simulink library "mixer_lib"  (Simulink 8.7)
settings: Solver=ode45  StartTime=0.0  StopTime=10.0  RelTol=1e-3
undefined symbols (not defined in the file): AdvDSPBChannelOutDisplay, DDC_CM_multiplication_factor, DDC_CM_NCO_phase, DDC_CM_NCO_sync, DDC_CM_number_of_bits_to_shift_left, DDC_LINEUP_param, dpoly, dspba_ChannelInVis, dspba_ChannelOutVis, dspba_internal_get_channel_ports, latency, value
libraries: DSPBAPrim x6, DSPBAWaveformSynth x2, DSPBABase x1
Description:
  | Digital Down Conversion 4 channel, 4 antenna reference design - complex mixer library
settings Model: Creator=bigcat  LastModifiedBy=5g

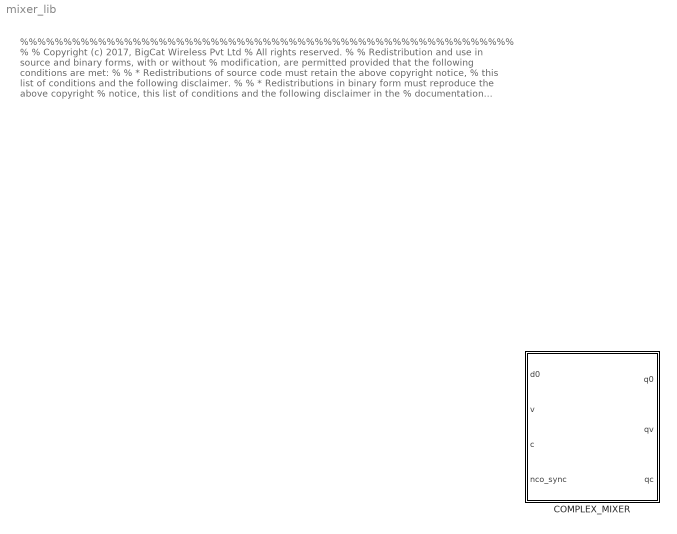
== system mixer_lib ==
  note: %%%%%%%%%%%%%%%%%%%%%%%%%%%%%%%%%%%%%%%%%%%%%%%%%%%%%%%%%
      |  %
      |  % Copyright (c) 2017, BigCat Wireless Pvt Ltd
      |  % All rights reserved.
      |  %
      |  % Redistribution and use in source and binary forms, with or without
      |  % modification, are permitted provided that the following conditions are met:
      |  %
      |  %     * Redistributions of source code must retain the above copyright notice,
      |  %       this list of conditions and the following disclaimer.
      |  %
      |  %     * Redistributions in binary form must reproduce the above copyright
      |  %       notice, this list of conditions and the following disclaimer in the
      |  %       documentation and/or other materials provided with the distribution.
      |  %
      |  %     * Neither the name of the copyright holder nor the names of its contributors
      |  %       may be used to endorse or promote products derived from this software
      |  %       without specific prior written permission.
      |  %
      |  %
      |  %
      |  % THIS SOFTWARE IS PROVIDED BY THE COPYRIGHT HOLDERS AND CONTRIBUTORS "AS IS"
      |  % AND ANY EXPRESS OR IMPLIED WARRANTIES, INCLUDING, BUT NOT LIMITED TO, THE
      |  % IMPLIED WARRANTIES OF MERCHANTABILITY AND FITNESS FOR A PARTICULAR PURPOSE ARE
      |  % DISCLAIMED. IN NO EVENT SHALL THE COPYRIGHT HOLDER OR CONTRIBUTORS BE LIABLE
      |  % FOR ANY DIRECT, INDIRECT, INCIDENTAL, SPECIAL, EXEMPLARY, OR CONSEQUENTIAL
      |  % DAMAGES (INCLUDING, BUT NOT LIMITED TO, PROCUREMENT OF SUBSTITUTE GOODS OR
      |  % SERVICES; LOSS OF USE, DATA, OR PROFITS; OR BUSINESS INTERRUPTION) HOWEVER
      |  % CAUSED AND ON ANY THEORY OF LIABILITY, WHETHER IN CONTRACT, STRICT LIABILITY,
      |  % OR TORT (INCLUDING NEGLIGENCE OR OTHERWISE) ARISING IN ANY WAY OUT OF THE USE
      |  % OF THIS SOFTWARE, EVEN IF ADVISED OF THE POSSIBILITY OF SUCH DAMAGE.
      |  %
      |   %%%%%%%%%%%%%%%%%%%%%%%%%%%%%%%%%%%%%%%%%%%%%%%%%%%%%%%%%%
  COMPLEX_MIXER : Subsystem  mask{CM_clock_margin=DDC_LINEUP_param.ClockMargin, CM_NCO_sample_rate=DDC_LINEUP_param.Complex_NCO.sample_rate, CM_NCO_accumulator_bit_width=DDC_LINEUP_param.Complex_NCO.accum_bit_width, CM_NCO_frequency_word=DDC_LINEUP_param.Complex_NCO.freq_word, CM_NCO_base_addr=DDC_LINEUP_param.Complex_NCO.base_addr, CM_NCO_data_type=DDC_LINEUP_param.Complex_NCO.data_type, CM_NCO_scaling_value=DDC_LINEUP_param.Complex_NCO.scaling_value, CM_sample_rate=DDC_LINEUP_param.CM.SampleRate, CM_complex_channels=DDC_LINEUP_param.CM.num_complex_chans, CM_complex_freq=DDC_LINEUP_param.CM.num_complex_freqs, CM_output_word_length=DDC_LINEUP_param.output_word_length, CM_output_fraction_length=DDC_LINEUP_param.output_fraction_length, CM_scale_multiplication_factor=DDC_CM_multiplication_factor, CM_scale_left_shift_factor=DDC_CM_number_of_bits_to_shift_left, CM_NCO_phase=DDC_CM_NCO_phase, CM_NCO_sync=DDC_CM_NCO_sync}
      mask prompts: CM_clock_margin "Clock margin"; CM_NCO_sample_rate "NCO sample rate"; CM_NCO_accumulator_bit_width "NCO accumulator bit width"; CM_NCO_frequency_word "NCO Frequency word"; CM_NCO_base_addr "NCO base address"; CM_NCO_data_type "NCO data type"; CM_NCO_scaling_value "NCO scaling value"; CM_sample_rate "Sample Rate"; CM_complex_channels "Number of complex channels"; CM_complex_freq "Number of complex frequencies"; CM_output_word_length "Output word length"; CM_output_fraction_length "Output fraction length"; CM_scale_multiplication_factor "Scale multiplication factor"; CM_scale_left_shift_factor "Scale left-shift factor"; CM_NCO_phase "NCO phase"; CM_NCO_sync "NCO sync"
      mask Display:
      | disp('COMPLEX\nMIXER');
      | port_label('input',1,'d0');
      | port_label('input',2,'v');
      | port_label('input',3,'c');
      | port_label('input',4,'nco_sync');
      | port_label('output',1,'q0');
      | port_label('output',2,'qv');
      | port_label('output',3,'qc');

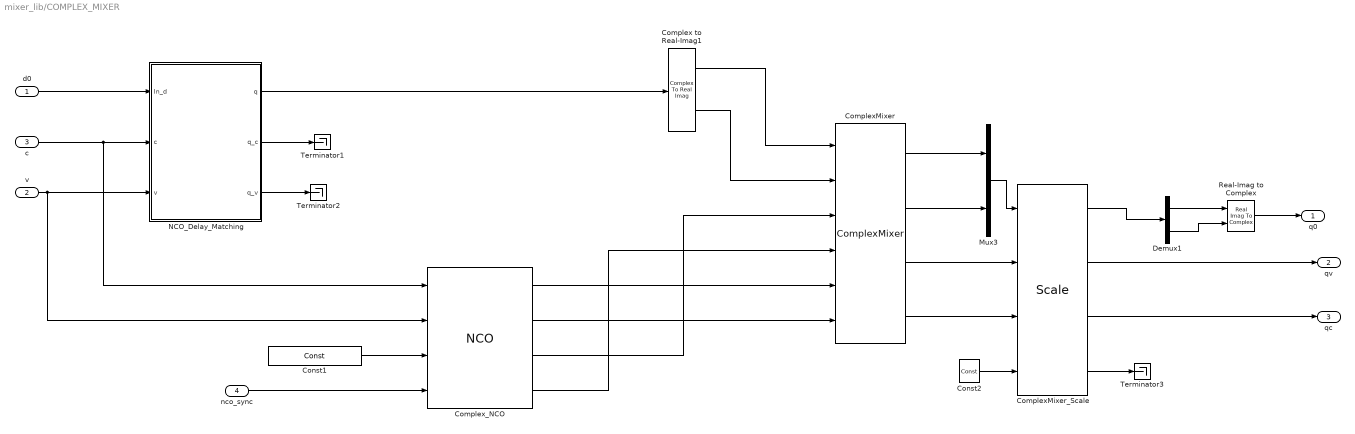
== system mixer_lib/COMPLEX_MIXER ==
  d0 : Inport
  v : Inport  Port=2
  c : Inport  Port=3
  nco_sync : Inport  Port=4
  Complex to Real-Imag1 : ComplexToRealImag
  ComplexMixer : DSPBAWaveformSynth/ComplexMixer  nInputRate=CM_sample_rate  nchan=CM_complex_channels  nfreq=CM_complex_freq  latency=4  version=20090407
  ComplexMixer_Scale : DSPBABase/Scale  otype=sfix(CM_output_word_length)  scale=2^-CM_output_fraction_length  rndmethod=Truncate  factor=CM_scale_multiplication_factor  satmethod=None  shift_vec=CM_scale_left_shift_factor  latency=0  wideSimulation=off  version=20130807
  Complex_NCO : DSPBAWaveformSynth/NCO  outputRate=CM_NCO_sample_rate  otype=sfix(CM_NCO_data_type)  scale=2^-CM_NCO_scaling_value  expSFDR=96.32  accumBitWidth=CM_NCO_accumulator_bit_width  accumPrecision=+/- 3.6621  phaseIncrAndInv=CM_NCO_frequency_word  phaseIncrInMHz="[0  0  0  0  0  0  0  0]"  phaseIncrAndInvMap=CM_NCO_base_addr  rwmode=Read/Write  exposebus=off  outWidth=5  tableSize=8  latency=18  version=20090407
      settings: AttributesFormatString=%<latency>
  Const1 : DSPBAPrim/Const  primtype=const  nInputs=0  nOutputs=1  omode=Specify via dialog  otype=ufix(24)  scale=2^-0  rndmethod=Unbiased  factor=1  satmethod=Symmetric  shift_vec=[0 1 2 -1]  value=CM_NCO_phase  inPortNames=['+'; '+';]  outPortNames=[' ']  dspbaimage=dspba_prim.jpg  text=fprintf('%s', num2str(value));  style=Optimised  visibilities=8 + 1024  floatPrecision=float32_m23  version=20120820
  Const2 : DSPBAPrim/Const  primtype=const  nInputs=0  nOutputs=1  omode=Specify via dialog  otype=ufix(1)  scale=1  rndmethod=Unbiased  factor=1  satmethod=Symmetric  shift_vec=[0 1 2 -1]  value=0  inPortNames=['+'; '+';]  outPortNames=[' ']  dspbaimage=dspba_prim.jpg  text=fprintf('%s', num2str(value));  style=Optimised  visibilities=8 + 1024  floatPrecision=float32_m23  version=20120820
  Demux1 : Demux  Outputs=2
  Mux3 : Mux  Inputs=2
  "NCO_Delay_Matching " : Subsystem
  Real-Imag to Complex : RealImagToComplex
  Terminator1 : Terminator
  Terminator2 : Terminator
  Terminator3 : Terminator
  q0 : Outport
  qv : Outport  Port=2
  qc : Outport  Port=3
  wires:
  Demux1/2 -> Real-Imag to Complex/2
  Demux1/1 -> Real-Imag to Complex/1
  ComplexMixer_Scale/4 -> Terminator3/1
  Const2/1 -> ComplexMixer_Scale/4
  Complex_NCO/1 -> ComplexMixer/5
  Complex_NCO/2 -> ComplexMixer/6
  ComplexMixer_Scale/3 -> qc/1
  ComplexMixer_Scale/2 -> qv/1
  ComplexMixer/1 -> Mux3/1
  ComplexMixer/2 -> Mux3/2
  Mux3/1 -> ComplexMixer_Scale/1
  ComplexMixer/4 -> ComplexMixer_Scale/3
  ComplexMixer/3 -> ComplexMixer_Scale/2
  Const1/1 -> Complex_NCO/3
  Real-Imag to Complex/1 -> q0/1
  ComplexMixer_Scale/1 -> Demux1/1
  Complex to Real-Imag1/1 -> ComplexMixer/1
  Complex_NCO/4 -> ComplexMixer/4
  Complex_NCO/3 -> ComplexMixer/3
  Complex to Real-Imag1/2 -> ComplexMixer/2
  "NCO_Delay_Matching "/1(q) -> Complex to Real-Imag1/1
  "NCO_Delay_Matching "/2(q_c) -> Terminator1/1
  "NCO_Delay_Matching "/3(q_v) -> Terminator2/1
  d0/1 -> "NCO_Delay_Matching "/1(In_d)
  c/1 -> Complex_NCO/1, "NCO_Delay_Matching "/2(c)
  v/1 -> Complex_NCO/2, "NCO_Delay_Matching "/3(v)
  nco_sync/1 -> Complex_NCO/4

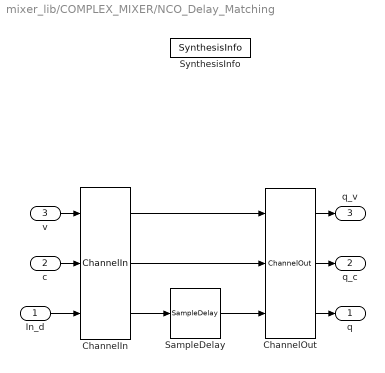
== system mixer_lib/COMPLEX_MIXER/NCO_Delay_Matching  ==
  In_d : Inport
  c : Inport  Port=2
  v : Inport  Port=3
  ChannelIn : DSPBAPrim/ChannelIn  primtype=channelin  nInputs=dspba_internal_get_channel_ports(gcb)  nOutputs=dspba_internal_get_channel_ports(gcb)  omode=Inherit via internal rule  otype=sfix(16)  scale=2^-15  rndmethod=Unbiased  factor=1  satmethod=Symmetric  shift_vec=[0 1 2 -1]  value=1  inPortNames=['v'; 'c'; '0'; '1'; '2'; '3'; '4'; '5'; '6'; '7'; '8'; '9'; 'A'; 'B'; 'D'; 'E'; 'F'; 'G'; 'H'; 'I'; 'J'; 'K'; 'L'; 'M'; 'N'; 'O'; 'P'; 'Q'; 'R'; 'S'; 'T'; 'U'; 'W'; 'X'; 'Y'; 'Z']  outPortNames=['v'; 'c'; '0'; '1'; '2'; '3'; '4'; '5'; '6'; '7'; '8'; '9'; 'A'; 'B'; 'D'; 'E'; 'F'; 'G'; 'H'; 'I'; 'J'; 'K'; 'L'; 'M'; 'N'; 'O'; 'P'; 'Q'; 'R'; 'S'; 'T'; 'U'; 'W'; 'X'; 'Y'; 'Z']  dspbaimage=dspba_prim.jpg  text=fprintf('In');  style=Optimised  dataSignals=1  foldingEnabled=off  channels=1  sampleRate=200  packetBeginPresent=off  packetBeginEnabled=off  visibilities=dspba_ChannelInVis(gcb)  latencyCorrection=0  version=20141013
  ChannelOut : DSPBAPrim/ChannelOut  primtype=channelout  nInputs=dspba_internal_get_channel_ports(gcb)  nOutputs=dspba_internal_get_channel_ports(gcb)  omode=Inherit via internal rule  otype=sfix(16)  scale=2^-15  rndmethod=Unbiased  factor=1  satmethod=Symmetric  shift_vec=[0 1 2 -1]  value=1  inPortNames=['v'; 'c'; '0'; '1'; '2'; '3'; '4'; '5'; '6'; '7'; '8'; '9'; 'A'; 'B'; 'D'; 'E'; 'F'; 'G'; 'H'; 'I'; 'J'; 'K'; 'L'; 'M'; 'N'; 'O'; 'P'; 'Q'; 'R'; 'S'; 'T'; 'U'; 'W'; 'X'; 'Y'; 'Z']  outPortNames=['v'; 'c'; '0'; '1'; '2'; '3'; '4'; '5'; '6'; '7'; '8'; '9'; 'A'; 'B'; 'D'; 'E'; 'F'; 'G'; 'H'; 'I'; 'J'; 'K'; 'L'; 'M'; 'N'; 'O'; 'P'; 'Q'; 'R'; 'S'; 'T'; 'U'; 'W'; 'X'; 'Y'; 'Z']  dspbaimage=dspba_prim.jpg  text=fprintf('Out%s', AdvDSPBChannelOutDisplay(latency));  style=Optimised  dataSignals=1  foldingEnabled=off  channels=1  sampleRate=200  packetBeginPresent=off  packetBeginEnabled=off  visibilities=dspba_ChannelOutVis(gcb)  latency=0  latencyCorrection=0  version=20141013
  SampleDelay : DSPBAPrim/SampleDelay  primtype=sampdelay  nInputs=1  nOutputs=1  omode=Inherit via internal rule  otype=sfix(16)  scale=2^-15  rndmethod=Unbiased  factor=1  satmethod=Symmetric  shift_vec=[0 1 2 -1]  value=2  inPortNames=[' '; ' ';]  outPortNames=[' ']  dspbaimage=dspba_prim.jpg  text=dpoly(1, eye(1,value+1), 'z')  style=Optimised  visibilities=8 + 1024 + 2^17 + 2^18  flexible=off  slackgroup=0  augmented=0  version=20090407  advOptions=[]
  SynthesisInfo : DSPBAPrim/SynthesisInfo  primtype=synthinfo  nInputs=0  nOutputs=0  omode=Inherit via internal rule  otype=sfix(16)  scale=2^-15  rndmethod=Truncate  factor=1  satmethod=Symmetric  shift_vec=[0 1 2 -1]  value=99  inPortNames=[' '; ' ';]  outPortNames=[' ']  dspbaimage=dspba_prim_ctrl.jpg  text=fprintf('Style=%s', style);  style=Scheduled  visibilities=2^17+2^18+2^19+2^20  constraintInUse=on  constraintRelation==  constraintLimit=2  bitAccurate=off  version=20150220
  q : Outport
  q_c : Outport  Port=2
  q_v : Outport  Port=3
  wires:
  ChannelIn/3 -> SampleDelay/1
  ChannelIn/2 -> ChannelOut/2
  ChannelIn/1 -> ChannelOut/1
  c/1 -> ChannelIn/2
  v/1 -> ChannelIn/1
  In_d/1 -> ChannelIn/3
  ChannelOut/2 -> q_c/1
  ChannelOut/1 -> q_v/1
  ChannelOut/3 -> q/1
  SampleDelay/1 -> ChannelOut/3
